simulink model "e2e"  (R2021a)
settings: Solver=VariableStepAuto  StartTime=0.0  StopTime=10.0  RelTol=1e-3
libraries: visionsources x1
settings Model: Creator=pranshu  LastModifiedBy=pranshu

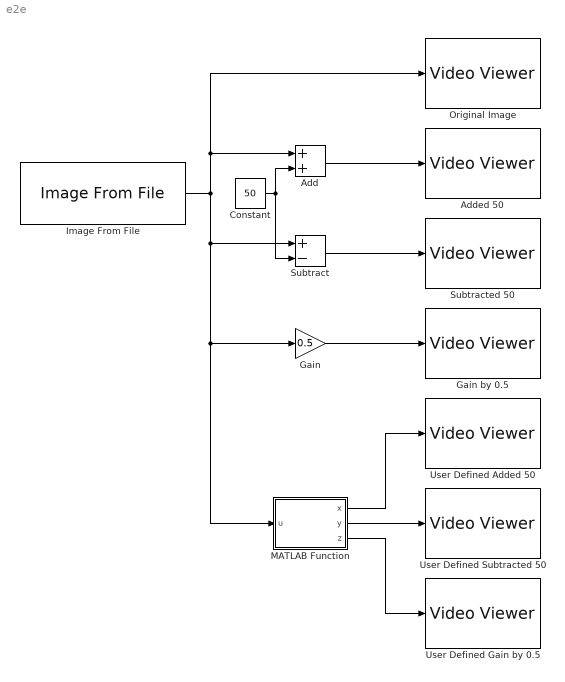
== system e2e ==
  Add : Sum  SaturateOnIntegerOverflow=on
  Added 50 : VideoViewer  FigPos=[93.8 462 417.6 304]
  Constant : Constant  Value=50  OutDataTypeStr=uint8
  Gain : Gain  Gain=0.5  OutDataTypeStr=uint8  SaturateOnIntegerOverflow=on
  Gain by 0.5 : VideoViewer  FigPos=[957 779.6 417.6 304]
  Image From File : visionsources/Image From File  Tag=vipblks_nd  FileName=cameraman.tif  Ts=inf  imagePorts=One multidimensional signal  OutPortLabels=R|G|B  ImageDataType=Inherit from input image  sdImageDataType=uint(8)  Signed=on  WordLength=16  FractionLengthMode=User-defined  FractionLength=15
  MATLAB Function : MATLAB Function  TreatAsAtomicUnit=on
  Original Image : VideoViewer  FigPos=[105 570.8 417.6 304]
  Subtract : Sum  Inputs=+-  SaturateOnIntegerOverflow=on
  Subtracted 50 : VideoViewer  FigPos=[1041 551.6 417.6 304]
  User Defined Added 50 : VideoViewer  FigPos=[559 583 418 304]
  User Defined Gain by 0.5 : VideoViewer  FigPos=[559 583 418 304]
  User Defined Subtracted 50 : VideoViewer  FigPos=[648.2 570.8 417.6 304]
  wires:
  Constant/1 -> Subtract/2, Add/2
  Image From File/1 -> Subtract/1, Gain/1, MATLAB Function/1(u), Add/1, Original Image/1
  Subtract/1 -> Subtracted 50/1
  Add/1 -> Added 50/1
  Gain/1 -> Gain by 0.5/1
  MATLAB Function/2(y) -> User Defined Subtracted 50/1
  MATLAB Function/1(x) -> User Defined Added 50/1
  MATLAB Function/3(z) -> User Defined Gain by 0.5/1

== matlab function e2e/MATLAB Function ==
  data: x output; u input; y output; z output
function [x,y,z] = fcn(u)
x=u+50;
y=u-50;
z=u*0.5;
